simulink model "La1b_open"  (R2024b)
settings: Solver=VariableStepAuto  StartTime=0.0  StopTime=100.0  RelTol=1e-3
values from neighbouring files (symbols this model uses):
  b = 666.1*10^-6    (= 0.0006661)    [Lab1b.m]
  J = 0.0081    [Lab1b.m]
  K_t = 0.094    [Lab1b.m]
  La = 528e-6    (= 0.000528)    [Lab1b.m]
  Ra = 0.649    [Lab1b.m]
settings Model: Creator=camer  LastModifiedBy=camer

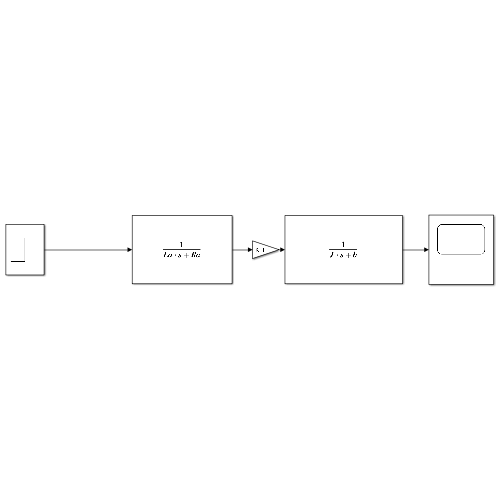
[thumbnail: Simulink's stored preview of the top-level diagram]
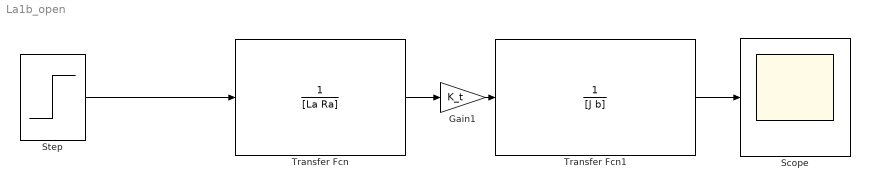
== system La1b_open ==
  Gain1 : Gain  Gain=K_t
  Scope : Scope
  Step : Step  After=60  SampleTime=0
  Transfer Fcn : TransferFcn  Denominator=[La Ra]
  Transfer Fcn1 : TransferFcn  Denominator=[J b]
  wires:
  Transfer Fcn1/1 -> Scope/1
  Step/1 -> Transfer Fcn/1
  Gain1/1 -> Transfer Fcn1/1
  Transfer Fcn/1 -> Gain1/1
